simulink model "Model_Sim_of_regulator"  (R2023b)
settings: Solver=ode4  StartTime=0.0  StopTime=Sim_time  FixedStep=Sampling_time  RelTol=1e-3
values from neighbouring files (symbols this model uses):
  c = 1    [Primary system response time.m]    (also in Primary_system_response_time.m; SET_Sim_of_State_deviation_FB_PD.m = 2; SET_Sim_of_State_deviation_FB_P_D.m = 2; SET_Sim_of_integral_servo_I_PD.m = 2)
  K = -place(A,B,p)    [SET_Sim_of_regulator_control.m]    (also in SET_Simulation_of_regulator_control.m)
  k = 10    [SET_Sim_of_State_deviation_FB_PD.m]    (also in SET_Sim_of_State_deviation_FB_P_D.m = 1; SET_Sim_of_integral_servo_I_PD.m; SET_Sim_of_regulator_control.m; SET_Sim_of_state_deviation_FB_and_output_integral_PID.m)
  m = 1    [SET_Sim_of_State_deviation_FB_PD.m]    (also in SET_Sim_of_State_deviation_FB_P_D.m; SET_Sim_of_integral_servo_I_PD.m; SET_Sim_of_regulator_control.m; SET_Sim_of_state_deviation_FB_and_output_integral_PID.m)
  Sampling_time = 0.001    [SET_Sim_of_State_deviation_FB_PD.m]    (also in SET_Sim_of_State_deviation_FB_P_D.m; SET_Sim_of_integral_servo_I_PD.m; SET_Sim_of_regulator_control.m; SET_Sim_of_state_deviation_FB_and_output_integral_PID.m)
  x0 = q0    [Primary system response time.m]    (also in Primary_system_response_time.m; SET_Sim_of_State_deviation_FB_PD.m = zeros(2,1); SET_Sim_of_State_deviation_FB_P_D.m = zeros(2,1); SET_Sim_of_integral_servo_I_PD.m = zeros(2,1))
settings Model: Creator=yuyas  LastModifiedBy=yuyas
settings DataIOCC: ReturnWorkspaceOutputs=off

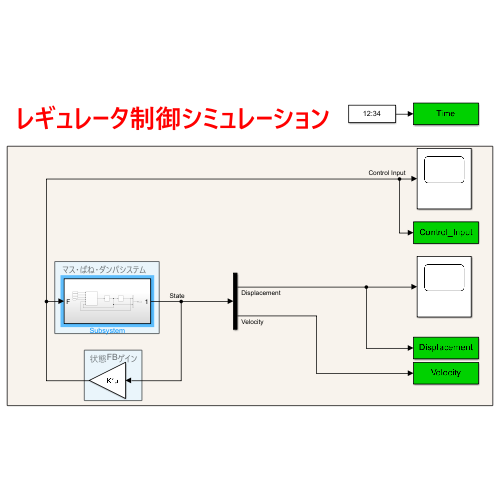
[thumbnail: Simulink's stored preview of the top-level diagram]
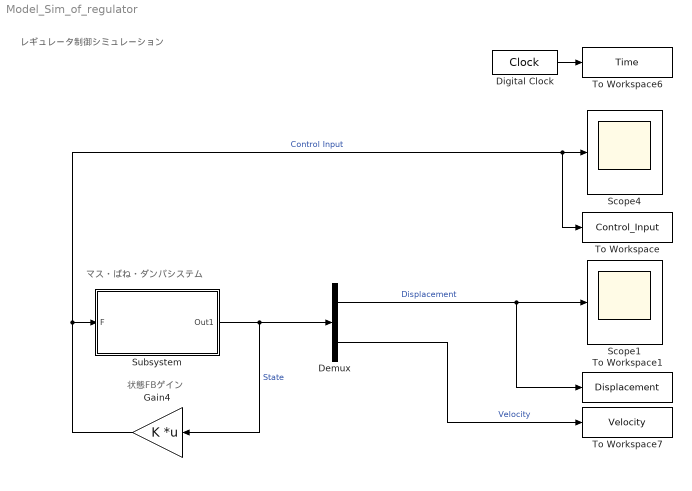
== system Model_Sim_of_regulator ==
  note: レギュレータ制御シミュレーション
  note: 状態FBゲイン
  note: マス・ばね・ダンパシステム
  Demux : Demux  Outputs=2
  Digital Clock : DigitalClock  SampleTime=Sampling_time
  Gain4 : Gain  Gain=K  Multiplication=Matrix(K*u)
  Scope1 : Scope
  Scope4 : Scope
  Subsystem : Subsystem
  To Workspace : ToWorkspace  VariableName=Control_Input  SampleTime=-1
      settings: Save2DSignal=2-D array (concatenate along first dimension)
  To Workspace1 : ToWorkspace  VariableName=Displacement  SampleTime=-1
      settings: Save2DSignal=2-D array (concatenate along first dimension)
  To Workspace6 : ToWorkspace  VariableName=Time  SampleTime=-1
      settings: Save2DSignal=2-D array (concatenate along first dimension)
  To Workspace7 : ToWorkspace  VariableName=Velocity  SampleTime=-1
      settings: Save2DSignal=2-D array (concatenate along first dimension)
  wires:
  Gain4/1 -> To Workspace/1, Scope4/1, Subsystem/1(F)  "Control Input"
  Subsystem/1(Out1) -> Gain4/1, Demux/1  "State"
  Demux/2 -> To Workspace7/1  "Velocity"
  Demux/1 -> Scope1/1, To Workspace1/1  "Displacement"
  Digital Clock/1 -> To Workspace6/1

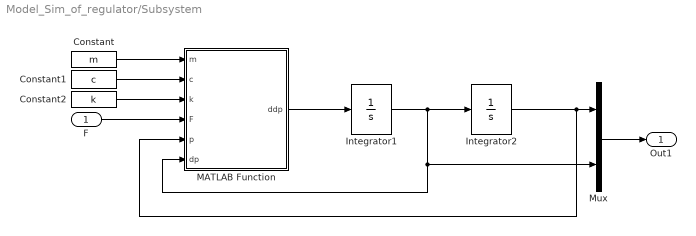
== system Model_Sim_of_regulator/Subsystem ==
  F : Inport
  Constant : Constant  Value=m
  Constant1 : Constant  Value=c
  Constant2 : Constant  Value=k
  Integrator1 : Integrator  InitialCondition=x0(2,1)
  Integrator2 : Integrator  InitialCondition=x0(1,1)
  MATLAB Function : MATLAB Function  TreatAsAtomicUnit=on
  Mux : Mux  Inputs=2
  Out1 : Outport  PortDimensions=2
  wires:
  MATLAB Function/1(ddp) -> Integrator1/1
  F/1 -> MATLAB Function/4(F)
  Mux/1 -> Out1/1
  Constant/1 -> MATLAB Function/1(m)
  Constant1/1 -> MATLAB Function/2(c)
  Constant2/1 -> MATLAB Function/3(k)
  Integrator1/1 -> Integrator2/1, Mux/2, MATLAB Function/6(dp)
  Integrator2/1 -> MATLAB Function/5(p), Mux/1

== matlab function Model_Sim_of_regulator/Subsystem/MATLAB Function ==
  data: m input; c input; k input; F input; ddp output; p input; dp input
function ddp = fcn(m, c, k, F,p,dp)

ddp = (-c/m)*dp+(-c/m)*p+(1/m)*F;

end
